simulink model "stellaris_lp_irreceive_RC5"  (R2017a)
settings: Solver=FixedStepDiscrete  StartTime=0.0  StopTime=0.5  FixedStep=ts  RelTol=1e-3  EnableMultiTasking=on
undefined symbols (not defined in the file or in its folder): ts
libraries: simulink x5, stellaris_lp_lib x4
settings Model: ExtModeTrigDuration=2  Creator=peselnikmg  LastModifiedBy=Nilim
settings DataIOCC: LimitDataPoints=on  SaveFormat=Array  SignalLoggingSaveFormat=ModelDataLogs  ReturnWorkspaceOutputs=on
settings OptimizationCC: UseDivisionForNetSlopeComputation=on  UseFloatMulNetSlope=on  UseSpecifiedMinMax=on  PassReuseOutputArgsAs=Individual arguments  ExpressionDepthLimit=2147483647  ZeroExternalMemoryAtStartup=off  ZeroInternalMemoryAtStartup=off  NoFixptDivByZeroProtection=on  EfficientFloat2IntCast=on  LifeSpan=inf  MaxStackSize=64  OptimizeBlockOrder=speed
settings DebuggingCC: ReadBeforeWriteMsg=DisableAll  WriteAfterWriteMsg=DisableAll  WriteAfterReadMsg=DisableAll  MultiTaskDSMMsg=none  IntegerOverflowMsg=error  ParameterTunabilityLossMsg=error  FcnCallInpInsideContextMsg=warning  AssertControl=DisableAll  StateNameClashWarn=warning  NonBusSignalsTreatedAsBus=error  SFInvalidInputDataAccessInChartInitDiag=error  SFTransitionOutsideNaturalParentDiag=error  SFUnreachableExecutionPathDiag=error  SFUndirectedBroadcastEventsDiag=error  SFExecutionAtInitializationDiag=none  IntegerSaturationMsg=error
settings HardwareCC: ProdBitPerPointer=32  ProdBitPerSizeT=32  ProdBitPerPtrDiffT=32  ProdLargestAtomicInteger=Long  ProdLargestAtomicFloat=Double  ProdWordSize=32  ProdHWDeviceType=ARM Compatible->ARM Cortex
settings ModelReferenceCC: UpdateModelReferenceTargets=IfOutOfDate  PropagateSignalLabelsOutOfModel=off
settings SFSimCC: SFSimEcho=off  MATLABDynamicMemAlloc=off
settings RTWCC: SystemTargetFile=ert.tlc  HardwareBoard=Tiva TM4C123G Launchpad  TLCOptions=-aInlineSetEventsForThisBaseRateFcn=TLC_FALSE -aSuppressMultiTaskScheduler=TLC_FALSE -aRateBasedStepFcn=1  TemplateMakefile=ert_default_tmf  Description=Embedded Coder  GenerateReport=on  RTWVerbose=off  Toolchain=Texas Instruments Code Composer Studio (Tiva)  BuildConfiguration=Faster Runs  IncludeHyperlinkInReport=on  LaunchReport=on  GenerateTraceInfo=on  GenerateTraceReport=on  GenerateTraceReportSl=on  GenerateTraceReportSf=on  GenerateTraceReportEml=on
settings CodeAppCC: ForceParamTrailComments=on  IgnoreCustomStorageClasses=off  OperatorAnnotations=on  SimulinkDataObjDesc=on  SFDataObjDesc=on  MATLABFcnDesc=on  CustomSymbolStrType=$N$R$M  InsertBlockDesc=on  MATLABSourceComments=on  EnableCustomComments=on  ReqsInCode=on
settings ERTTargetCC: UtilityFuncGeneration=Shared location  CombineSignalStateStructs=on  SuppressErrorStatus=on  SupportNonFinite=off  ParenthesesLevel=Maximum  CastingMode=Standards  EnableSignedLeftShifts=off  EnableSignedRightShifts=off
settings ConfigComp: CovMetricSettings=dw  CovHtmlReporting=on  CovSaveCumulativeToWorkspaceVar=on  CovSaveSingleToWorkspaceVar=on  CovExternalEMLEnable=off

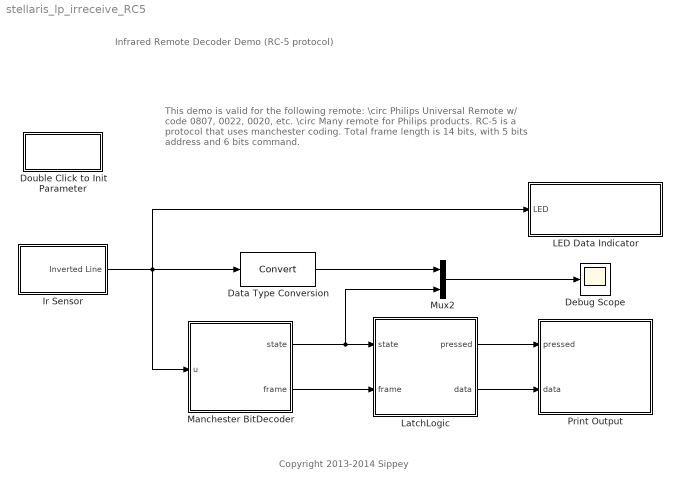
== system stellaris_lp_irreceive_RC5 ==
  note: This demo is valid for the following remote:
      | \circ  Philips Universal Remote w/ code 0807, 0022, 0020, etc.
      | \circ  Many remote for Philips products.
      |
      | RC-5 is a protocol that uses manchester coding. Total frame length
      | is 14 bits, with 5 bits address and 6 bits command.
  note: Infrared Remote Decoder Demo (RC-5 protocol)
  note: Copyright 2013-2014 Sippey
  Data Type Conversion : DataTypeConversion  SampleTime=ts
  Debug Scope : Scope
  Double Click to Init Parameter : Subsystem
      settings: OpenFcn=ts=0.0001;
      mask Display: fprintf('Double-click');
  Ir Sensor : Subsystem
  LED Data Indicator : Subsystem
  LatchLogic : Stateflow chart  TreatAsAtomicUnit=on
  Manchester BitDecoder : Stateflow chart  TreatAsAtomicUnit=on
  Mux2 : Mux  Inputs=2
  Print Output : Subsystem
  wires:
  Mux2/1 -> Debug Scope/1
  Ir Sensor/1(Inverted Line) -> Manchester BitDecoder/1(u), Data Type Conversion/1, LED Data Indicator/1(LED)
  Data Type Conversion/1 -> Mux2/1
  LatchLogic/1(pressed) -> Print Output/1(pressed)
  LatchLogic/2(data) -> Print Output/2(data)
  Manchester BitDecoder/1(state) -> Mux2/2, LatchLogic/1(state)
  Manchester BitDecoder/2(frame) -> LatchLogic/2(frame)

== system stellaris_lp_irreceive_RC5/Double Click to Init Parameter ==

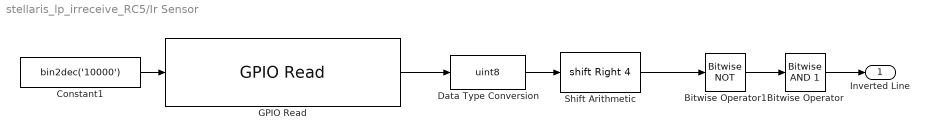
== system stellaris_lp_irreceive_RC5/Ir Sensor ==
  Bitwise Operator : simulink/Logic and Bit Operations/Bitwise Operator  logicop=AND  UseBitMask=on  BitMask=1  BitMaskRealWorld=Stored Integer
  Bitwise Operator1 : simulink/Logic and Bit Operations/Bitwise Operator  logicop=NOT  UseBitMask=off  BitMask=1  BitMaskRealWorld=Stored Integer
  Constant1 : Constant  Value=bin2dec('10000')  OutDataTypeStr=Inherit: Inherit via back propagation
  Data Type Conversion : DataTypeConversion  OutDataTypeStr=uint8  SampleTime=ts
  GPIO Read : stellaris_lp_lib/GPIO/GPIO Read  GPIO_PORTX_BASE=GPIO_PORTF_BASE  SampleTime=-1
      settings: SourceProductName=Run on Stellaris LaunchPad
  Shift Arithmetic : ArithShift  BitShiftNumber=4  BitShiftDirection=Right
  Inverted Line : Outport
  wires:
  Constant1/1 -> GPIO Read/1
  Shift Arithmetic/1 -> Bitwise Operator1/1
  GPIO Read/1 -> Data Type Conversion/1
  Bitwise Operator1/1 -> Bitwise Operator/1
  Bitwise Operator/1 -> Inverted Line/1
  Data Type Conversion/1 -> Shift Arithmetic/1

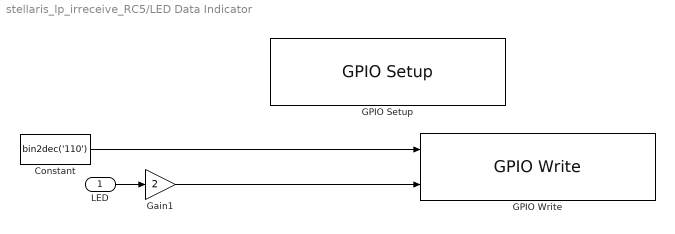
== system stellaris_lp_irreceive_RC5/LED Data Indicator ==
  LED : Inport
  Constant : Constant  Value=bin2dec('110')  OutDataTypeStr=Inherit: Inherit via back propagation
  GPIO Setup : stellaris_lp_lib/GPIO/GPIO Setup  GPIO_PORTX_BASE=GPIO_PORTF_BASE  PinsOutput_0=Input  PinsOutput_1=Output  PinsOutput_2=Output  PinsOutput_3=Output  PinsOutput_4=Input  PinsOutput_5=Input  PinsOutput_6=Input  PinsOutput_7=Input
      settings: SourceProductName=Run on Stellaris LaunchPad
  GPIO Write : stellaris_lp_lib/GPIO/GPIO Write  GPIO_PORTX_BASE=GPIO_PORTF_BASE  SampleTime=-1
      settings: SourceProductName=Run on Stellaris LaunchPad
  Gain1 : Gain  Gain=2  OutDataTypeStr=Inherit: Inherit via back propagation
  wires:
  Constant/1 -> GPIO Write/1
  Gain1/1 -> GPIO Write/2
  LED/1 -> Gain1/1

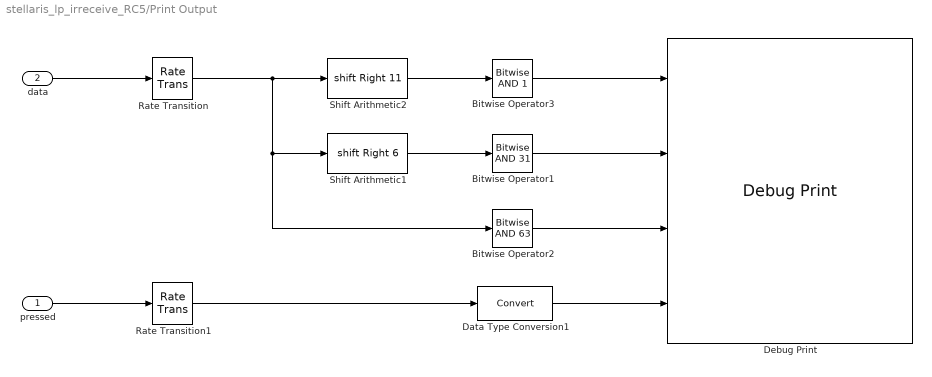
== system stellaris_lp_irreceive_RC5/Print Output ==
  pressed : Inport
  data : Inport  Port=2
  Bitwise Operator1 : simulink/Logic and Bit Operations/Bitwise Operator  logicop=AND  UseBitMask=on  BitMask=31  BitMaskRealWorld=Stored Integer
  Bitwise Operator2 : simulink/Logic and Bit Operations/Bitwise Operator  logicop=AND  UseBitMask=on  BitMask=63  BitMaskRealWorld=Stored Integer
  Bitwise Operator3 : simulink/Logic and Bit Operations/Bitwise Operator  logicop=AND  UseBitMask=on  BitMask=1  BitMaskRealWorld=Stored Integer
  Data Type Conversion1 : DataTypeConversion
  Debug Print : stellaris_lp_lib/Debug/Debug Print  fmt='toggle: %d, addr: %02X, key %d, pressed %d'  sample_time=0.1
      settings: SourceProductName=Run on Stellaris LaunchPad
  Rate Transition : RateTransition
  Rate Transition1 : RateTransition
  Shift Arithmetic1 : ArithShift  BitShiftNumber=6  BitShiftDirection=Right
  Shift Arithmetic2 : ArithShift  BitShiftNumber=11  BitShiftDirection=Right
  wires:
  Rate Transition/1 -> Shift Arithmetic2/1, Bitwise Operator2/1, Shift Arithmetic1/1
  Shift Arithmetic1/1 -> Bitwise Operator1/1
  Rate Transition1/1 -> Data Type Conversion1/1
  data/1 -> Rate Transition/1
  pressed/1 -> Rate Transition1/1
  Shift Arithmetic2/1 -> Bitwise Operator3/1
  Data Type Conversion1/1 -> Debug Print/4
  Bitwise Operator3/1 -> Debug Print/1
  Bitwise Operator1/1 -> Debug Print/2
  Bitwise Operator2/1 -> Debug Print/3

== stateflow chart stellaris_lp_irreceive_RC5/LatchLogic ==
  state NotPressed
    pressed=0;
    data=0;
  state Pressed
    pressed=1;
  note: If repeat stub is seen, the bit decoder will go
      | to the BitDecoded state once and then timeout.
      | Reset the temporal logic at this time.
  note: timeout after 150ms
      | if a repeat msg have
      | not show up yet
  (default) -> NotPressed
  NotPressed -> Pressed : [state==1]{data=frame;}
  Pressed -> Pressed [order 2] : [state==1]
  Pressed -> NotPressed [order 1] : after(0.15,sec)
  data: state input int32 =0; frame input int32; pressed output int32; data output int32

== stateflow chart stellaris_lp_irreceive_RC5/Manchester BitDecoder ==
  state Idle
    state = -1;
    nb=0;
  state Output
    state=1;
  state start1
    state = -3;
  state mid1
    state = -2;
    nb=nb+1;
  note: timeout
  note: 14 bits frame:
      | 2 start bits
      | 1 toggle bit
      | 5 address bits
      | 6 command bits
  note: pulse/space length
      | 	long: ~1.8ms   (01/10 bit back to back)
      | 	short: ~0.9 ms  (individual bit transition)
      | Let 1.4 ms be the threshold
  state start0
    state = -5;
  state mid0
    state = -4;
    nb=nb+1;
  note: reference: http://www.clearwater.com.au/code/rc5
  (default) -> Idle
  Output -> Idle
  (junction 272) -> Idle : after(5e-3,sec)
  start1 -> Output [order 3] : [nb>=14]
  mid0 -> Output [order 4] : [nb>=14]
  Idle -> mid1 : [u==1]{frame=1;}
  start1 -> mid1 [order 1] : before(1.4e-3,sec)[u==1]
      | {frame=2*frame+1;}
  mid1 -> start1 [order 2] : before(1.4e-3, sec)[u==0]
  start1 -> (junction 272) [order 2]
  mid1 -> (junction 272) [order 3]
  mid0 -> mid1 [order 1] : after(1.4e-3, sec)[u==1]
      | {frame=2*frame+1;}
  mid1 -> mid0 [order 1] : after(1.4e-3, sec)[u==0]
      | {frame=2*frame;}
  mid0 -> (junction 272) [order 3]
  start0 -> (junction 272) [order 2]
  start0 -> mid0 [order 1] : before(1.4e-3,sec)[u==0]
      | {frame=2*frame;}
  mid0 -> start0 [order 2] : before(1.4e-3, sec)[u==1]
  data: u input; state output int32 =0; nb local int32; frame output int32
